simulink model "dev_sim_lineal_kalman_v2"  (R2019b)
settings: Solver=VariableStepAuto  StartTime=0.0  StopTime=100.0  RelTol=1e-3
values from neighbouring files (symbols this model uses):
  A_0 = eval(A_0)    [modelo.m]    (also in modelo_var.m; parametros.mat = [0 -3.26931291643 0 0.71460251427 0 0 0 0 1 -0.0325743287495)
  B_0 = eval(B_0)    [modelo.m]    (also in modelo_var.m; parametros.mat = [0 0 0 0 0 0 1190.47619048 0 0 0 0 0 ... (16 elements, 8x2)])
  C_0 = eval(C_0)    [modelo.m]    (also in modelo_var.m; parametros.mat = [1 0 0 0 0 1 0 0 0 0 0 0 ... (16 elements, 2x8)])
  D_0 = eval(D_0)    [modelo.m]    (also in modelo_var.m; parametros.mat = [0  0; 0  0])
  R = R2*R1    [modelo.m]    (also in modelo_var.m = eye(2))
undefined symbols (not defined in the file or in its folder): Continuous, Time
libraries: ctrlSharedLib x1
settings Model: Creator=tronc  LastModifiedBy=tronc

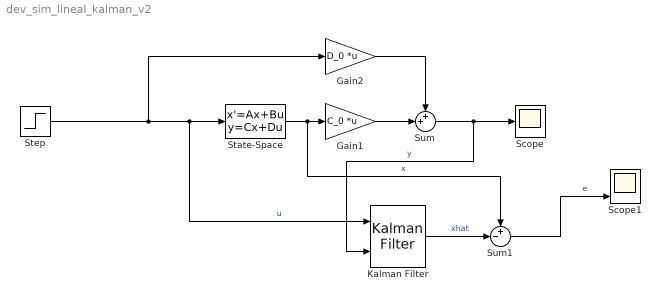
== system dev_sim_lineal_kalman_v2 ==
  Gain1 : Gain  Gain=C_0  Multiplication=Matrix(K*u)
  Gain2 : Gain  Gain=D_0  Multiplication=Matrix(K*u)
  Kalman Filter : ctrlSharedLib/Kalman Filter  TimeDomain=Continuous-Time  UseCurrentEstimator=on  ModelSource=Individual A, B, C, D matrices  ModelSourceVariable=ss(0.95,1,1,0,1)  A=A_0  B=B_0  C=C_0  D=D_0  NumberOfStates=1  NumberOfInputs=1  NumberOfOutputs=1  InitialEstimateSource=Dialog  X0=[0 0 0 0 0 0 0 0]  P0=10  UseK=off  UseGH=off  NumberOfProcessNoiseInputs=1  G=1  TimeInvariantG=on  H=0  TimeInvariantH=on  Q=Q  TimeInvariantQ=on  R=R  TimeInvariantR=on  N=0  TimeInvariantN=on  AddInputPort=on  AddEnablePort=off  OutputEstimatedY=off  OutputP=off  Ts=-1
      settings: SourceProductBaseCode=CT
  Scope : Scope
  Scope1 : Scope  NumInputPorts=3
  State-Space : StateSpace  A=A_0  B=B_0  C=eye(8)  D=zeros(8,2)  InitialCondition=[1 1 0 0 0 0 0 0]
  Step : Step  Before=[0 0]  After=[1 1]  SampleTime=0
  Sum : Sum  Inputs=++|
  Sum1 : Sum  Inputs=+-|
  wires:
  State-Space/1 -> Sum1/1, Gain1/1  "x"
  Step/1 -> Gain2/1, Kalman Filter/1, State-Space/1  "u"
  Sum/1 -> Kalman Filter/2, Scope/1  "y"
  Gain2/1 -> Sum/1
  Gain1/1 -> Sum/2
  Kalman Filter/1 -> Sum1/2  "xhat"
  Sum1/1 -> Scope1/3  "e"
